simulink library "XsensLibrary"  (R2014b)
settings: Solver=ode45  StartTime=0.0  StopTime=10.0  RelTol=1e-3
settings Model: Creator=philipp  LastModifiedBy=control

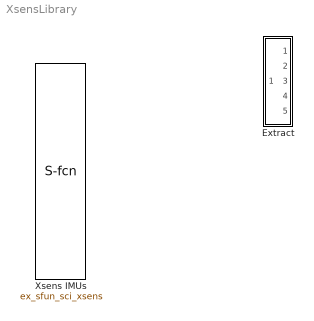
== system XsensLibrary ==
  Extract : Subsystem  mask{correction=off}
      mask prompts: correction "Use correction"
      mask DialogControl Control2 Prompt: Correction means that when N packets get lost, the value of a and omega is divided by N. (The Xsens Library adds up all increments, thus when a packet is not received it will be added to the next one)
      mask Display:
      | port_label('output', 1, 'a', 'texmode', 'on'),
      | port_label('output', 2, '\omega', 'texmode', 'on'),
      | port_label('output', 3, 'mag', 'texmode', 'on'),
      | port_label('output', 4, 'q', 'texmode', 'on'),
      | port_label('output', 5, 'sig', 'texmode', 'on'),
  Xsens IMUs : S-Function  FunctionName=ex_sfun_sci_xsens  Parameters=uint8(SID00)', uint8(SID01)', uint8(SID02)', uint8(SID03)', uint8(SID04)', uint8(SID05)', uint8(SID06)', uint8(SID07)', uint8(SID08)', uint8(SID09)', uint8(SID10)', uint32(Freq), uint32(UseCalibratedValues), Ts  EnableBusSupport=off  mask{SID00='/dev/xsens_dongle_1', SID01='00340454', SID02='0', SID03='0', SID04='/dev/xsens_mtx_405783', SID05='/dev/xsens_mtx_405784', SID06='0', SID07='0', SID08='0', SID09='0', SID10='0', Freq=100, Ts=0.01, UseCalibratedValues=on}
      mask prompts: SID00 "WirelessMasterSerialPort"; SID01 "SensorId/SerialPort"; SID02 "SensorId/SerialPort"; SID03 "SensorId/SerialPort"; SID04 "SensorId/SerialPort"; SID05 "SensorId/SerialPort"; SID06 "SensorId/SerialPort"; SID07 "SensorId/SerialPort"; SID08 "SensorId/SerialPort"; SID09 "SensorId/SerialPort"; SID10 "SensorId/SerialPort"; Freq "Frequency"; Ts "Block Sampling Interval Ts"; UseCalibratedValues "Use calibrated values provided by Xsens"
      mask DialogControl DescTextVar Prompt: This block is for connecting the wireless Xsens IMUs MTw via the Xsens USB dongle or the Xsens docking station.
      mask DialogControl Control3 Prompt: Sensor ID: The IDs of the connected Sensors. Init will wait for all listed sensor IDs!
      mask DialogControl Control2 Prompt: Frequency: The sampling frequency of the individual IMUs. The frequency can be chosen higher than the block sampling rate. In this case, multiple IMU data packets can be available available at the output
      mask DialogControl Control4 Prompt: Use calibrated values: In this case, the acceleration and the angular velocity will not be derived by increments of the raw data but by a complex algorithm provided by Xsens
      mask Display:
      | text(0.02,0.5,'Xsens'),
      | port_label('output', 1, 'S01'),
      | port_label('output', 2, 'S02'),
      | port_label('output', 3, 'S03'),
      | port_label('output', 4, 'S04'),
      | port_label('output', 5, 'S05'),
      | port_label('output', 6, 'S06'),
      | port_label('output', 7, 'S07'),
      | port_label('output', 8, 'S08'),
      | port_label('output', 9, 'S09'),
      | port_label('output', 10, 'S10'),

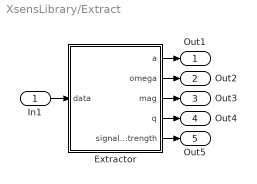
== system XsensLibrary/Extract ==
  In1 : Inport
  Extractor : MATLAB Function  TreatAsAtomicUnit=on
  Out1 : Outport
  Out2 : Outport  Port=2
  Out3 : Outport  Port=3
  Out4 : Outport  Port=4
  Out5 : Outport  Port=5
  wires:
  In1/1 -> Extractor/1(data)
  Extractor/5(signalStrength) -> Out5/1
  Extractor/3(mag) -> Out3/1
  Extractor/4(q) -> Out4/1
  Extractor/2(omega) -> Out2/1
  Extractor/1(a) -> Out1/1

== matlab function XsensLibrary/Extract/Extractor ==
  data: data input; a output; omega output; mag output; q output; signalStrength output; correction parameter
function [a, omega, mag, q, signalStrength] = fcn(data, correction)
%#codegen

newestDataSet = data(1:16);

sampleNumber   = newestDataSet(1);
a_raw          = newestDataSet(2:4);
omega_raw      = newestDataSet(5:7);
mag_raw        = newestDataSet(8:10);
q_raw          = newestDataSet(11:14);
signalStrength = newestDataSet(15);
unknown        = newestDataSet(16);


persistent lastSampleNumber lastFactor

if isempty(lastSampleNumber)
    lastSampleNumber = 0;
    lastFactor = 1;
end

factor = 1;

diff = abs(sampleNumber - lastSampleNumber);

if diff >= 1
    factor = diff;
end
if diff == 0
    factor = lastFactor;
end

lastFactor = factor;
lastSampleNumber = sampleNumber;

if correction == 1
    a = a_raw/factor;
    omega = omega_raw/factor;
    mag = mag_raw;
    q = q_raw;
else
    a = a_raw;
    omega = omega_raw;
    mag = mag_raw;
    q = q_raw;
end
